simulink model "WashMachine"  (R2020b)
settings: Solver=VariableStepAuto  StartTime=0.0  StopTime=10.0  RelTol=1e-3
settings Model: Creator=apple  LastModifiedBy=apple

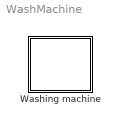
== system WashMachine ==
  Washing machine : Stateflow chart  TreatAsAtomicUnit=on

== stateflow chart WashMachine/Washing machine ==
  state OFF
    state Initial_State
    state off
      en:time = 0;
      finish = 0;
    state Pending_State
    (default) -> off
    off -> Initial_State : ON
    Pending_State -> off [order 2] : OFF
  state ON
    on E:fprintf("Washing Completed!");
    (history)
    state Add_Water
      du:time = time + 1;
    state Washing
      du:time = time + 1;
    Add_Water -> Washing : [time >= n1]/{time = 0;}
    Washing -> Add_Water : [time >= n2]/{time = 0;}
  (default) -> OFF
  Initial_State -> Add_Water : SWITCH
  ON -> OFF [order 1] : OFF
  ON -> OFF [order 3] : after(n3,sec)[finish == 0]{finish = 1;send(E);}
  Pending_State -> ON [order 1] : SWITCH
  ON -> Pending_State [order 2] : SWITCH{n3 = n3 - temporalCount(sec)}
  data: n1 local =5; n2 local =10; n3 local =45; finish local; time local
  events: E local FUNCTION_CALL_EVENT; SWITCH local RISING_EDGE_EVENT; ON local FUNCTION_CALL_EVENT; OFF local FUNCTION_CALL_EVENT
